simulink model "UxAxGen"  (Simulink 7.7)
settings: Solver=ode3  StartTime=0  StopTime=500  FixedStep=1  RelTol=1e-3
InitFcn:
  | dir = pwd;
  | mex desiredUxAx.c
  | m = 1650;
  | a = 1.04;
  | b = 1.42;
  | h = .75;
  | load seg_prm;
  | load map_prm;
  | load cumSum;
values from neighbouring files (symbols this model uses):
  cumSum = [77.319195 200.525496 374.723026 475.995466 523.118866 586.011313 627.725335 700.969343 756.097147 757.127347 796.364692 827.061539 ... (64 elements, 64x1)]    [cumSum.mat]    (also in cumSumDavid.mat = [73.081465 117.575783 232.945004 282.160803 305.410289 387.7)
  map_prm = [0 0 0 0 0 64 0 0]    [map_prm.mat]    (also in map_prmDavid.mat = [0 0 0 0 0 83 0 0])
  seg_prm = [0 1 2 3 4 5 6 7 8 9 10 11 ... (832 elements, 64x13)]    [seg_prm.mat]    (also in seg_prmDavid.mat = [0 1 2 3 4 5 6 7 8 9 10 11 ... (1079 elements, 83x13)])
settings Model: Creator=ddl  LastModifiedBy=nkapania

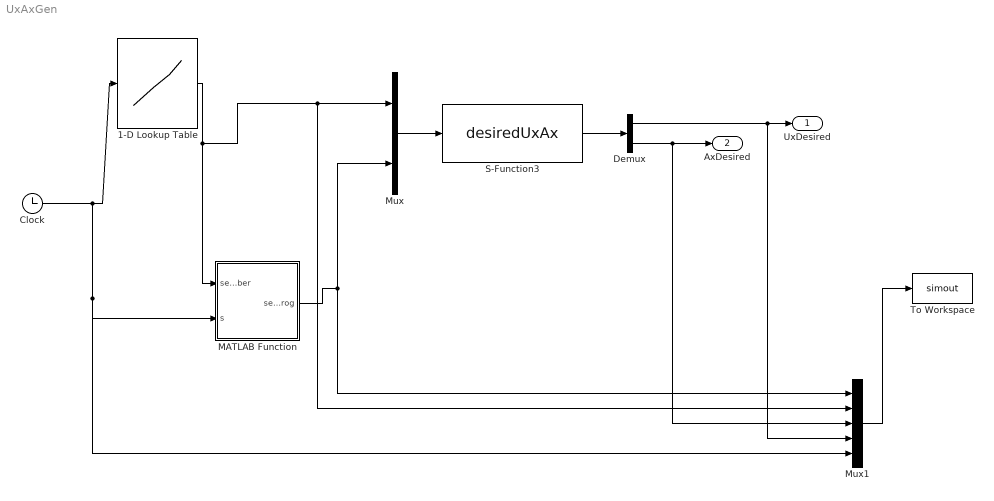
== system UxAxGen ==
  1-D Lookup Table : Lookup_n-D  NumberOfTableDimensions=1  BreakpointsForDimension1=[0; cumSum]  Table=[0; [1:1:64]']  InterpMethod=Flat  ExtrapMethod=Clip  DiagnosticForOutOfRangeInput=Error  UseLastTableValue=on  InputSameDT=on
  Clock : Clock
      settings: Decimation=10
  Demux : Demux  Outputs=2
  MATLAB Function : Stateflow chart  TreatAsAtomicUnit=on
  Mux : Mux  Inputs=2
  Mux1 : Mux  Inputs=5
  S-Function3 : S-Function  FunctionName=desiredUxAx  Parameters=m,a,b,h,map_prm,seg_prm  EnableBusSupport=off
  To Workspace : ToWorkspace  VariableName=simout  SampleTime=-1  SaveFormat=Array
  UxDesired : Outport
  AxDesired : Outport  Port=2
  wires:
  Mux/1 -> S-Function3/1
  S-Function3/1 -> Demux/1
  Demux/1 -> UxDesired/1, Mux1/4
  Demux/2 -> Mux1/3, AxDesired/1
  Clock/1 -> 1-D Lookup Table/1, MATLAB Function/2(s), Mux1/5
  MATLAB Function/1(segProg) -> Mux/2, Mux1/1
  1-D Lookup Table/1 -> MATLAB Function/1(segNumber), Mux/1, Mux1/2
  Mux1/1 -> To Workspace/1

== matlab function MATLAB Function ==
  data: segNumber input double; segProg output double; s input double; cumSum parameter double
function segProg = fcn(segNumber, s, cumSum)
%#codegen

if segNumber == 0
    segProg = s;
else
    segProg = s - cumSum(segNumber);
end
